simulink model "SOLAR_GRIDleadacidbattery"  (R2021a)
settings: Solver=VariableStepAuto  StartTime=0.0  StopTime=5  RelTol=1e-3
undefined symbols (not defined in the file): Acid, C_boost, D1, Delta, L_boost, Lead, sigbuilder_block
libraries: spsSeriesRLCBranchLib x9, spsVoltageMeasurementLib x4, spsBreakerLib x3, spsCurrentMeasurementLib x3, spsDiodeLib x2, spsIGBTDiodeLib x2, spsPWMGeneratorDCDCLib x2, spsThreePhaseVIMeasurementLib x2, spsBatteryLib x1, spsPVArrayLib x1, spsGroundLib x1, spsPWMGenerator2LevelLib x1
settings Model: Creator=Dell  LastModifiedBy=Dell

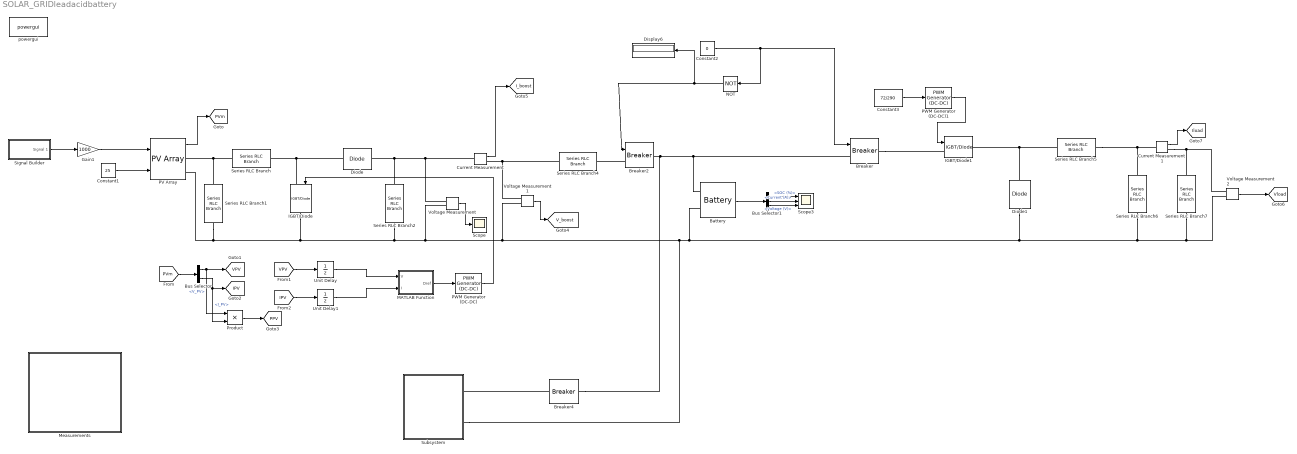
== system SOLAR_GRIDleadacidbattery ==
  Battery : spsBatteryLib/Battery  BatType=Lead-Acid  ShowTempParam=off  ThermalPreset=no  ShowAgeParam=off  NomV=290  NomQ=150  SOC=50  Batt_Tr=1  PresetModel=on  MaxQ=156.25  MinV=217.5  FullV=315.7566  Dis_rate=30  R=0.019333  Normal_OP=46.5417  expZone="[295.2467           0.5]"  current=[6.5 13 32.5]  Units=Time  Tci=20  NomT=20  T2=-30  MaxQ2=4.8  FullV2=7.1  Normal_OP2=5.655  expZone2="[6.58           1]"  Rca=0.6  ti=2000  Dp=0  Neq0=0  Tsim=1e6  Ta1=25  Qeol=5.4*0.9  Reol=0.013333*1.2  Char_age=[2.3478, 3]  Dis_age=[2.3478, 10]  N1=1500  N2=10500  N3=1000  N4=1400  Ta2=45  N5=950
  Breaker : spsBreakerLib/Breaker  InitialState=0  SwitchingTimes=[3]  External=on  BreakerResistance=0.01  SnubberResistance=1e6  SnubberCapacitance=inf  Measurements=None  MoreParameters=on  NoBreakLoop=off
      settings: SourceProductBaseCode=PS
  Breaker2 : spsBreakerLib/Breaker  InitialState=0  SwitchingTimes=[3]  External=on  BreakerResistance=0.01  SnubberResistance=1e6  SnubberCapacitance=inf  Measurements=None  MoreParameters=on  NoBreakLoop=off
      settings: SourceProductBaseCode=PS
  Breaker4 : spsBreakerLib/Breaker  InitialState=0  SwitchingTimes=[2 3,4 5]  External=off  BreakerResistance=0.01  SnubberResistance=1e6  SnubberCapacitance=inf  Measurements=None  MoreParameters=on  NoBreakLoop=off
      settings: SourceProductBaseCode=PS
  Bus Selector : BusSelector  OutputSignals=V_PV,I_PV
  Bus Selector1 : BusSelector  OutputSignals=SOC (%),Current (A),Voltage (V)
  Constant1 : Constant  Value=25
  Constant2 : Constant  Value=0
  Constant3 : Constant  Value=72/290
  Current Measurement : spsCurrentMeasurementLib/Current Measurement  PhasorSimulation=off  OutputType=Complex  PSBequivalent=0
  Current Measurement1 : spsCurrentMeasurementLib/Current Measurement  PhasorSimulation=off  OutputType=Complex  PSBequivalent=0
  Diode : spsDiodeLib/Diode  Ron=0.001  Lon=0  Vf=0.8  IC=0  UseSnubber=0  Rs=500  Cs=250e-9  Measurements=off
  Diode1 : spsDiodeLib/Diode  Ron=0.001  Lon=0  Vf=0.8  IC=0  UseSnubber=0  Rs=500  Cs=250e-9  Measurements=off
  Display6 : Display
  Gain1 : Gain  Gain=1000
  IGBT/Diode : spsIGBTDiodeLib/IGBT//Diode  Ron=1e-3  Rs=1e5  Cs=inf  Measurements=off
  IGBT/Diode1 : spsIGBTDiodeLib/IGBT//Diode  Ron=1e-3  Rs=1e5  Cs=inf  Measurements=off
  MATLAB Function : MATLAB Function  TreatAsAtomicUnit=on
  Measurements : Subsystem
  NOT : Logic  Operator=NOT  IconShape=distinctive  AllPortsSameDT=off  OutDataTypeStr=boolean
  PV Array : spsPVArrayLib/PV Array  Npar=9  Nser=7  PlotType=array @ 1000 W/m2 & specified temperatures  S_vec="[ 1000  500  100 ]"  Temp_C_vec="[ 45 25  ]"  ModuleName=User-defined  PlotWhenSelected=off  Pm=315  Ncell=72  Voc=45.8  Isc=8.92  Vm=37.5  Im=8.4  beta_Voc_pc=-0.36099  alpha_Isc_pc=0.102  beta_Voc=-0.16533  alpha_Isc=0.0090984  IL=8.9507  I0=3.3278e-10  nI=1.0316  Rsh=368.3938  Rs=0.3143  RobustModel=off  RobustCellTemperature=313.3991  BAL=on  Tc=1e-6  Tfilter=5e-5
  PWM Generator (DC-DC) : spsPWMGeneratorDCDCLib/PWM Generator (DC-DC)  Fsw=5000  Ts=0
  PWM Generator (DC-DC)1 : spsPWMGeneratorDCDCLib/PWM Generator (DC-DC)  Fsw=5000  Ts=0
  Product : Product
  Scope : Scope
  Scope3 : Scope  NumInputPorts=3
  Series RLC Branch : spsSeriesRLCBranchLib/Series RLC Branch  LConnTagsString=__new0  RConnTagsString=__new0  BranchType=L  Resistance=1  Inductance=L_boost  SetiL0=off  InitialCurrent=0  Capacitance=1e-6  Setx0=off  InitialVoltage=0  Measurements=None
  Series RLC Branch1 : spsSeriesRLCBranchLib/Series RLC Branch  LConnTagsString=__new0  RConnTagsString=__new0  BranchType=C  Resistance=1  Inductance=1e-3  SetiL0=off  InitialCurrent=0  Capacitance=1000e-6  Setx0=off  InitialVoltage=0  Measurements=None
  Series RLC Branch2 : spsSeriesRLCBranchLib/Series RLC Branch  LConnTagsString=__new0  RConnTagsString=__new0  BranchType=C  Resistance=1  Inductance=1e-3  SetiL0=off  InitialCurrent=0  Capacitance=C_boost  Setx0=off  InitialVoltage=0  Measurements=None
  Series RLC Branch4 : spsSeriesRLCBranchLib/Series RLC Branch  LConnTagsString=__new0  RConnTagsString=__new0  BranchType=L  Resistance=1  Inductance=1e-2  SetiL0=off  InitialCurrent=0  Capacitance=1e-6  Setx0=off  InitialVoltage=0  Measurements=None
  Series RLC Branch5 : spsSeriesRLCBranchLib/Series RLC Branch  LConnTagsString=__new0  RConnTagsString=__new0  BranchType=L  Resistance=1  Inductance=0.0078  SetiL0=off  InitialCurrent=0  Capacitance=1e-6  Setx0=off  InitialVoltage=0  Measurements=None
  Series RLC Branch6 : spsSeriesRLCBranchLib/Series RLC Branch  LConnTagsString=__new0  RConnTagsString=__new0  BranchType=RC  Resistance=10e-3  Inductance=1e-3  SetiL0=off  InitialCurrent=0  Capacitance=4.8225e-05  Setx0=off  InitialVoltage=0  Measurements=None
  Series RLC Branch7 : spsSeriesRLCBranchLib/Series RLC Branch  LConnTagsString=__new0  RConnTagsString=__new0  BranchType=R  Resistance=0.5184  Inductance=1e-3  SetiL0=off  InitialCurrent=0  Capacitance=1e-6  Setx0=off  InitialVoltage=0  Measurements=None
  Signal Builder : Subsystem  Tag=STV Subsys  LoadFcn=sigbuilder_block('load');  StartFcn=sigbuilder_block('start');  StopFcn=sigbuilder_block('stop');  ClipboardFcn=sigbuilder_block('clipboard');  mask(Sigbuilder block){tuvar=[0:10]}
      mask help: Simulink:masks:SigbuilderBlock_MD
      mask init:
      | if ~strcmp(get_param(bdroot(gcbh),'SimulationStatus'),'stopped') tuvar = sigbuilder_block('maskInit'); end
      settings: CopyFcn=sigbuilder_block('copy');  DeleteFcn=sigbuilder_block('delete');  ModelCloseFcn=sigbuilder_block('modelClose');  PreSaveFcn=sigbuilder_block('preSave');  PauseFcn=sigbuilder_block('pause');  ContinueFcn=sigbuilder_block('continue');  NameChangeFcn=sigbuilder_block('namechange');  OpenFcn=sigbuilder_block('open',[427.2 160.2 550.8 400.2 ]);  CloseFcn=sigbuilder_block('close');
      mask Display: plot(0, 0, 100, 100,[2, 2, 32, 32, 2], [68, 8, 8, 68, 68],[32, 2], [38, 38], [32, 19, 2],[53, 60, 44], [32, 17, 17, 2],[16, 16, 31, 31]);txt = getActiveGroup(gcbh);text(2, 100, txt,'verticalAlignment', 'top');
  Subsystem : Subsystem
  Unit Delay : UnitDelay  SampleTime=-1  HasFrameUpgradeWarning=on
  Unit Delay1 : UnitDelay  SampleTime=-1  HasFrameUpgradeWarning=on
  Voltage Measurement : spsVoltageMeasurementLib/Voltage Measurement  PhasorSimulation=off  OutputType=Complex  PSBequivalent=0
  Voltage Measurement1 : spsVoltageMeasurementLib/Voltage Measurement  PhasorSimulation=off  OutputType=Complex  PSBequivalent=0
  Voltage Measurement2 : spsVoltageMeasurementLib/Voltage Measurement  PhasorSimulation=off  OutputType=Complex  PSBequivalent=0
  powergui : spspowerguiLib/powergui  Priority=1  SimulationMode=Continuous  SampleTime=50e-6  frequency=60  Iterations=50  frequencyindice=0  Pbase=100e6  ErrMax=1e-4  UnitsV=kV  UnitsW=MW  buscounter=0  FunctionMessages=off  echomessages=off  EnableUseOfTLC=off  CurrentSourceSwitches=off  DisableSnubberDevices=off  DisableRonSwitches=off  DisableVfSwitches=off  DisplayEquations=off  AutomaticDiscreteSolvers=off  SolverType=Tustin/Backward Euler (TBE)  Interpol=off  ExternalGateDelay=off  methode=off  Ts=100  x0status=blocks  SPID=on  SwTol=0  HookPort=off  NonlinearTolerance=1e-4  nMaxIteration=100  ContinueOnMaxIteration=off  RestoreLinks=warning  ResistiveCurrentMeasurement=off  Frange=[0:2:500]  Ylog=off  Xlog=on  ShowGrid=off  save=off  variable=ZData  structure=0  ZoomFFT=off  StartTime=0.0  cycles=1  DisplayStyle=1  fundamental=60  FreqAxis=off  MaxFrequency=1000  frequencyindicesteady=1  RmsSteady=1  display=off
  tag scope: IPV=global, I_boost=global, Iload=global, PPV=global, PVm=global, VPV=global, V_boost=global, Vload=global
  wires:
  NOT/1 -> Display6/1, Breaker2/1
  Current Measurement1/1 -> [Iload]
  Constant2/1 -> NOT/1, Breaker/1
  Bus Selector1/3 -> Scope3/3  "<Voltage (V)>"
  Bus Selector/2 -> Product/2, [IPV]  "<I_PV>"
  Bus Selector1/1 -> Scope3/1  "<SOC (%)>"
  PWM Generator (DC-DC)1/1 -> IGBT/Diode1/1
  Constant3/1 -> PWM Generator (DC-DC)1/1
  [IPV] -> Unit Delay1/1
  MATLAB Function/1(Dref) -> PWM Generator (DC-DC)/1
  Battery/1 -> Bus Selector1/1
  Bus Selector1/2 -> Scope3/2  "<Current (A)>"
  PV Array/1 -> [PVm]
  Unit Delay/1 -> MATLAB Function/1(V)
  [PVm] -> Bus Selector/1
  [VPV] -> Unit Delay/1
  PWM Generator (DC-DC)/1 -> IGBT/Diode/1
  Bus Selector/1 -> [VPV], Product/1  "<V_PV>"
  Unit Delay1/1 -> MATLAB Function/2(I)
  Current Measurement/1 -> [I_boost]
  Constant1/1 -> PV Array/2
  Voltage Measurement/1 -> Scope/1
  Product/1 -> [PPV]
  Voltage Measurement1/1 -> [V_boost]
  Voltage Measurement2/1 -> [Vload]
  Gain1/1 -> PV Array/1
  Signal Builder/1(Signal 1) -> Gain1/1
  connections:
  Current Measurement/RConn1 -- Series RLC Branch4/LConn1 -- Voltage Measurement1/LConn1
  PV Array/RConn1 -- Series RLC Branch/LConn1 -- Series RLC Branch1/LConn1
  Voltage Measurement/LConn1 -- Series RLC Branch2/LConn1 -- Diode/RConn1 -- Current Measurement/LConn1
  Breaker/LConn1 -- Breaker4/RConn1 -- Breaker2/RConn1 -- Battery/LConn1
  Current Measurement1/RConn1 -- Series RLC Branch7/LConn1 -- Voltage Measurement2/LConn1
  Diode/LConn1 -- IGBT/Diode/LConn1 -- Series RLC Branch/RConn1
  IGBT/Diode1/RConn1 -- Diode1/RConn1 -- Series RLC Branch5/LConn1
  Series RLC Branch5/RConn1 -- Series RLC Branch6/LConn1 -- Current Measurement1/LConn1
  Breaker/RConn1 -- IGBT/Diode1/LConn1
  Breaker2/LConn1 -- Series RLC Branch4/RConn1
  Breaker4/LConn1 -- Subsystem/RConn1
  Series RLC Branch6/RConn1 -- Diode1/LConn1 -- Subsystem/RConn2 -- Voltage Measurement/LConn2 -- Series RLC Branch1/RConn1 -- PV Array/RConn2 -- IGBT/Diode/RConn1 -- Series RLC Branch2/RConn1 -- Voltage Measurement1/LConn2 -- Battery/LConn2 -- Series RLC Branch7/RConn1 -- Voltage Measurement2/LConn2

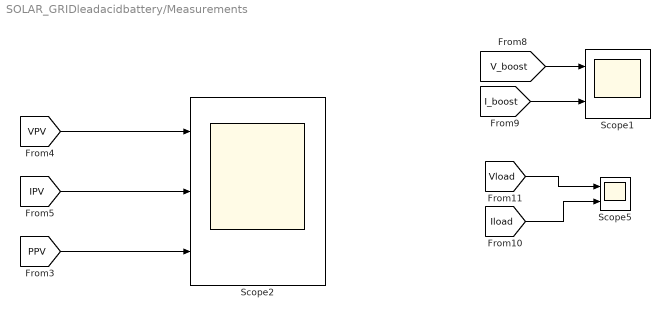
== system SOLAR_GRIDleadacidbattery/Measurements ==
  Scope1 : Scope  NumInputPorts=2
  Scope2 : Scope  NumInputPorts=3
  Scope5 : Scope  NumInputPorts=2
  wires:
  [V_boost] -> Scope1/1
  [Vload] -> Scope5/1
  [Iload] -> Scope5/2
  [I_boost] -> Scope1/2
  [PPV] -> Scope2/3
  [IPV] -> Scope2/2
  [VPV] -> Scope2/1

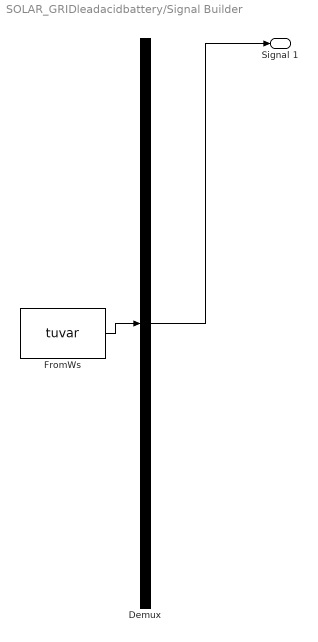
== system SOLAR_GRIDleadacidbattery/Signal Builder ==
  Demux : Demux  Tag=STV Demux  Outputs=1
      settings: DisplayOption=none
  FromWs : FromWorkspace  Tag=STV FromWs  VariableName=tuvar
      SigBuilderData=|
      | common.afterFinalStr = 'Extrapolate'
      | common.sampleTime = 0
      | dataSet.timeRange = [0 10]
      | dataSet.name = 'Group 1'
      | sbobj.Groups.Name = 'Group 1'
      | sbobj.Groups.Signals.Name = 'Signal 1'
      | sbobj.Groups.Signals.XData = [0 2 2 3 3 4.02 4.02 10]
      | sbobj.Groups.Signals.YData = [0.995 0.995 0 0 1.005 1 0 0]
  Signal 1 : Outport  Tag=STV Outport
  wires:
  Demux/1 -> Signal 1/1
  FromWs/1 -> Demux/1

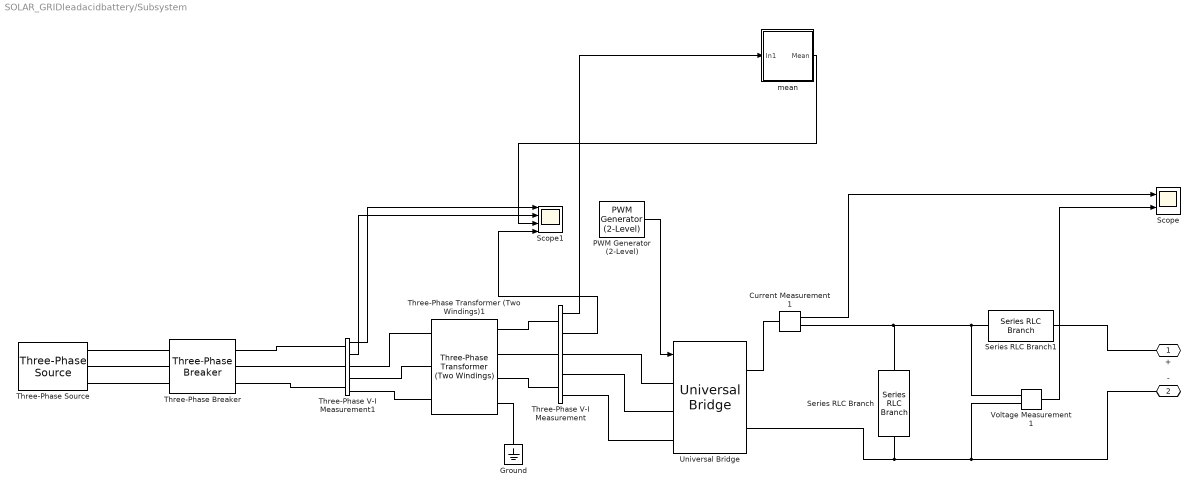
== system SOLAR_GRIDleadacidbattery/Subsystem ==
  Current Measurement1 : spsCurrentMeasurementLib/Current Measurement  PhasorSimulation=off  OutputType=Complex  PSBequivalent=0
  Ground : spsGroundLib/Ground  LConnTagsString=a
  PWM Generator (2-Level) : spsPWMGenerator2LevelLib/PWM Generator (2-Level)  ModulatorType=Three-phase bridge (6 pulses)  ModulatorMode=Unsynchronized  Fc=33*50  Pc=90  nF=27  MinMax="[ -1  1 ]"  SamplingTechnique=Natural  ModulatingSignals=on  m=0.8  Freq=50  Phase=0  Ts=0  ShowCarrierOutport=off
  Scope : Scope  NumInputPorts=2
  Scope1 : Scope  NumInputPorts=4
  Series RLC Branch : spsSeriesRLCBranchLib/Series RLC Branch  LConnTagsString=__new0  RConnTagsString=__new0  BranchType=C  Resistance=1  Inductance=1e-3  SetiL0=off  InitialCurrent=0  Capacitance=100e-4  Setx0=off  InitialVoltage=0  Measurements=None
  Series RLC Branch1 : spsSeriesRLCBranchLib/Series RLC Branch  LConnTagsString=__new0  RConnTagsString=__new0  BranchType=L  Resistance=1  Inductance=5e-2  SetiL0=off  InitialCurrent=0  Capacitance=100e-4  Setx0=off  InitialVoltage=0  Measurements=None
  Three-Phase Transformer (Two Windings)1 : spsThreePhaseTransformerTwoWindingsLib/Three-Phase Transformer (Two Windings)  Winding1Connection=Delta (D1)  Winding2Connection=Yn  CoreType=Three single-phase transformers  SetSaturation=off  Hysteresis=off  DataFile='hysteresis'  SetInitialFlux=off  Measurements=None  UNITS=pu  NominalPower=[25e3 , 50 ]  Winding1=[11e3 , 0.002 , 0.08 ]  Winding2=[240, 0.002 , 0.08 ]  Rm=500  Lm=500  L0=0.5  Saturation=[ 0,0 ; 0.0024,1.2 ; 1.0,1.52 ]  InitialFluxes=[ 0.8 , -0.8 , 0.7 ]  BreakLoop=off  DiscreteSolver=Trapezoidal iterative  DataType=off  TransfoNumber=1
  Three-Phase V-I Measurement : spsThreePhaseVIMeasurementLib/Three-Phase V-I Measurement  VoltageMeasurement=phase-to-phase  SetLabelV=off  LabelV=Vabc  Vpu=off  VpuLL=off  CurrentMeasurement=yes  SetLabelI=off  LabelI=Iabc  Ipu=off  Pbase=100e6  Vbase=500e3  OutputType=Complex  PhasorSimulation=off  PSBequivalent=0
  Three-Phase V-I Measurement1 : spsThreePhaseVIMeasurementLib/Three-Phase V-I Measurement  VoltageMeasurement=phase-to-phase  SetLabelV=off  LabelV=Vabc  Vpu=off  VpuLL=off  CurrentMeasurement=yes  SetLabelI=off  LabelI=Iabc  Ipu=off  Pbase=100e6  Vbase=500e3  OutputType=Complex  PhasorSimulation=off  PSBequivalent=0
  Three-Phase Breaker : spsThreePhaseBreakerLib/Three-Phase Breaker  InitialState=open  SwitchA=on  SwitchB=on  SwitchC=on  SwitchTimes=[2 3,4 5]  External=off  BreakerResistance=0.01  SnubberResistance=1e6  SnubberCapacitance=inf  Measurements=None
  Three-Phase Source : spsThreePhaseSourceLib/Three-Phase Source  InternalConnection=Yg  VoltagePhases=off  Voltage=11e3  PhaseAngle=0  Voltage_phases=[25e3 25e3 25e3]/sqrt(3)  PhaseAngles_phases=[0 -120 +120]  Frequency=50  NonIdealSource=on  SpecifyImpedance=off  Resistance=0.8929  Inductance=16.58e-3  ShortCircuitLevel=35e3  BaseVoltage=11e3  XRratio=7  BusType=swing  Pref=10e3  Qref=0  Prefabc=[10e3, 10e3, 10e3]  Qrefabc=[0, 0, 0]  Qmin=-inf  Qmax=inf
  Universal Bridge : spsUniversalBridgeLib/Universal Bridge  Arms=3  SnubberResistance=1e5  SnubberCapacitance=inf  Device=Thyristors  Ron=1e-3  Lon=0  ForwardVoltages="[  0  0  ]"  ForwardVoltage=0  GTOparameters=[ 10e-6 , 20e-6 ]  IGBTparameters=[ 1e-6 , 2e-6 ]  Measurements=None  Measurements_2=None  converterType=Rectifier
  Voltage Measurement1 : spsVoltageMeasurementLib/Voltage Measurement  PhasorSimulation=off  OutputType=Complex  PSBequivalent=0
  mean : Subsystem
  + : PMIOPort  Side=Right
  - : PMIOPort  Port=2  Side=Right
  wires:
  Voltage Measurement1/1 -> Scope/2
  Three-Phase V-I Measurement/2 -> Scope1/4
  mean/1(Mean) -> Scope1/3
  Three-Phase V-I Measurement1/1 -> Scope1/1
  PWM Generator (2-Level)/1 -> Universal Bridge/1
  Current Measurement1/1 -> Scope/1
  Three-Phase V-I Measurement/1 -> mean/1(In1)
  Three-Phase V-I Measurement1/2 -> Scope1/2
  connections:
  Universal Bridge/RConn2 -- -/RConn1 -- Voltage Measurement1/LConn2 -- Series RLC Branch/RConn1
  Voltage Measurement1/LConn1 -- Series RLC Branch1/LConn1 -- Current Measurement1/RConn1 -- Series RLC Branch/LConn1
  Current Measurement1/LConn1 -- Universal Bridge/RConn1
  Three-Phase Transformer (Two Windings)1/RConn2 -- Three-Phase V-I Measurement/LConn2
  Three-Phase Transformer (Two Windings)1/RConn1 -- Three-Phase V-I Measurement/LConn1
  Three-Phase V-I Measurement/RConn2 -- Universal Bridge/LConn2
  Three-Phase V-I Measurement/RConn1 -- Universal Bridge/LConn1
  Series RLC Branch1/RConn1 -- +/RConn1
  Three-Phase V-I Measurement/RConn3 -- Universal Bridge/LConn3
  Three-Phase V-I Measurement1/RConn2 -- Three-Phase Transformer (Two Windings)1/LConn2
  Three-Phase V-I Measurement1/RConn1 -- Three-Phase Transformer (Two Windings)1/LConn1
  Ground/LConn1 -- Three-Phase Transformer (Two Windings)1/RConn4
  Three-Phase V-I Measurement1/RConn3 -- Three-Phase Transformer (Two Windings)1/LConn3
  Three-Phase Transformer (Two Windings)1/RConn3 -- Three-Phase V-I Measurement/LConn3
  Three-Phase Breaker/LConn2 -- Three-Phase Source/RConn2
  Three-Phase Breaker/LConn1 -- Three-Phase Source/RConn1
  Three-Phase Breaker/LConn3 -- Three-Phase Source/RConn3
  Three-Phase Breaker/RConn1 -- Three-Phase V-I Measurement1/LConn1
  Three-Phase Breaker/RConn2 -- Three-Phase V-I Measurement1/LConn2
  Three-Phase Breaker/RConn3 -- Three-Phase V-I Measurement1/LConn3

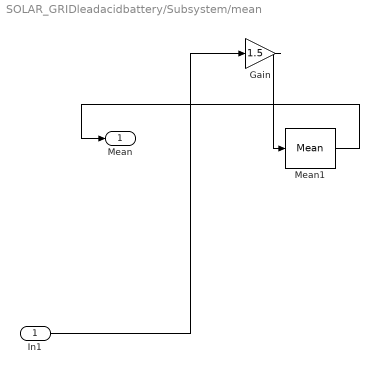
== system SOLAR_GRIDleadacidbattery/Subsystem/mean ==
  In1 : Inport
  Gain : Gain  Gain=1.5
  Mean1 : spsMeanLib/Mean  Freq=100  Vinit=0  Ts=0
  Mean : Outport
  wires:
  Mean1/1 -> Mean/1
  Gain/1 -> Mean1/1
  In1/1 -> Gain/1

== matlab function SOLAR_GRIDleadacidbattery/MATLAB Function ==
  data: V input; Dref output; I input
function Dref=MPPT(V,I)
duty_init = 0.1;
Dmin = 0.1;
Dmax = 0.9;
deldref=0.00008;
persistent Vold Pold Drefold;
if isempty(Vold)
    Vold=0;
    Pold=0;
    Drefold=duty_init;
end
P=V*I;
dV=V-Vold;
dP=P-Pold;
if dP~=0
    if dP<0
        if dV<0
            Dref=Drefold-deldref;
        else
            Dref=Drefold+deldref;
        end
    else
        if dV<0
            Dref=Drefold+deldref;
        else
            Dref=Drefold-deldref;
        end
    end
else
    Dref=Drefold;
end
if Dref>Dmax || Dref<Dmin
    Dref=Drefold;
end
Drefold=Dref;
Pold=P;
Vold=V;
